simulink model "LKWDaempfungsModell"  (R2019b)
settings: Solver=VariableStepAuto  StartTime=0.0  StopTime=15  RelTol=1e-5
values from neighbouring files (symbols this model uses):
  F_FederRuhe = m_Frachtraum * g    (= 22563)    [modelParameter.m]
  g = 9.81    [modelParameter.m]
  K_Feder = 98.1 *1000    (= 98100)    [modelParameter.m]
  m_Frachtraum = 2300    [modelParameter.m]
  MaxActuatorForce = 100 *1000    (= 100000)    [modelParameter.m]
  muh_daempfer = 3000    [modelParameter.m]
libraries: simulink x1
settings Model: Creator=du-wa  LastModifiedBy=du-wa

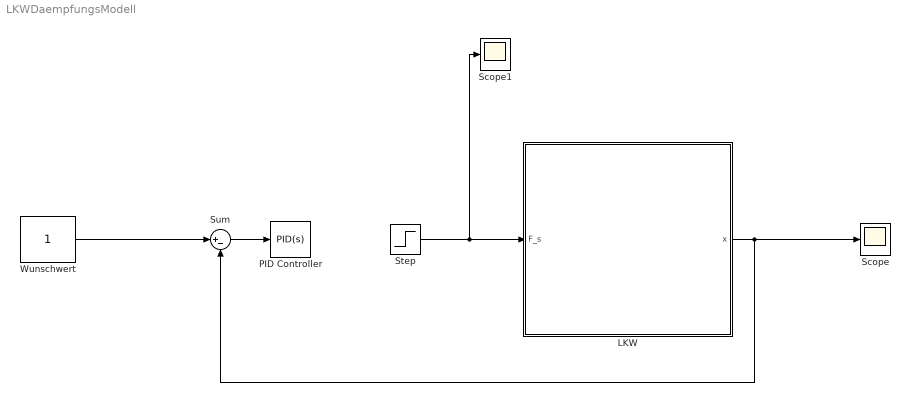
== system LKWDaempfungsModell ==
  "LKW " : Subsystem
  PID Controller : simulink/Continuous/PID Controller  Controller=PID  Form=Parallel  TimeDomain=Continuous-time  SampleTime=-1  IntegratorMethod=Forward Euler  FilterMethod=Forward Euler  ControllerParametersSource=internal  P=1000  I=1  D=0  UseFilter=on  N=100  TunerSelectOption=Transfer Function Based (PID Tuner App)  InitialConditionSource=internal  InitialConditionForIntegrator=0  InitialConditionForFilter=0  DifferentiatorICPrevScaledInput=0  ExternalReset=none  TrackingMode=off  Kt=1  LimitOutput=on  UpperSaturationLimit=MaxActuatorForce  LowerSaturationLimit=-MaxActuatorForce  LinearizeAsGain=on  AntiWindupMode=clamping  Kb=1  POutMin=[]  POutMax=[]  IOutMin=[]  IOutMax=[]  DOutMin=[]  DOutMax=[]  NOutMin=[]  NOutMax=[]  SumOutMin=[]  SumOutMax=[]  SaturationOutMin=[]  SaturationOutMax=[]  PParamMin=[]  PParamMax=[]  IParamMin=[]  IParamMax=[]  DParamMin=[]  DParamMax=[]  NParamMin=[]  NParamMax=[]  KbParamMin=[]  KbParamMax=[]  KtParamMin=[]  KtParamMax=[]  KbOutMin=[]  KbOutMax=[]  KtOutMin=[]  KtOutMax=[]  IntegratorOutMin=[]  IntegratorOutMax=[]  FilterOutMin=[]  FilterOutMax=[]  SumI1OutMin=[]  SumI1OutMax=[]  SumI2OutMin=[]  SumI2OutMax=[]  SumI3OutMin=[]  SumI3OutMax=[]  SumI4OutMin=[]  SumI4OutMax=[]  SumDOutMin=[]  SumDOutMax=[]  DifferentiatorOutMin=[]  DifferentiatorOutMax=[]  FilterDiffOutCoefMin=[]  FilterDiffOutCoefMax=[]  ReciprocalOutMin=[]  ReciprocalOutMax=[]  SumDenOutMin=[]  SumDenOutMax=[]  SumNumOutMin=[]  SumNumOutMax=[]  DivideOutMin=[]  DivideOutMax=[]  IntegratorContinuousStateAttributes=''  IntegratorStateMustResolveToSignalObject=off  IntegratorRTWStateStorageClass=Auto  FilterContinuousStateAttributes=''  FilterStateMustResolveToSignalObject=off  FilterRTWStateStorageClass=Auto  ParallelPVariant=InternalParameters  IdealPVariant=Disabled  IVariant=InternalParameters  DVariant=InternalParameters  IntegratorVariant=Continuous  SatVariant=Enabled  AWVariant=ContClampingParallel  PCopyVariant=Disabled  TRVariant=Disabled  FdbkBlocksVariant=Forward  IdealPFdbkVariant=Disabled  SatFdbkVariant=Disabled  DerivativeFilterVariant=ContFilter  NVariant=InternalParameters  NCopyVariant=Disabled  FilterICVariant=InternalICsFilter  IntegratorICVariant=InternalICs  ExternalResetVariant=Disabled  TRSumVariant=Passthrough  SumFdbkVariant=Disabled  SumVariant=Sum_PID
  Scope : Scope
  Scope1 : Scope
  Step : Step  After=1000  SampleTime=0
  Sum : Sum  Inputs=|+-
  Wunschwert : Constant
  wires:
  "LKW "/1(x) -> Scope/1, Sum/2
  Wunschwert/1 -> Sum/1
  Sum/1 -> PID Controller/1
  Step/1 -> Scope1/1, "LKW "/1(F_s)

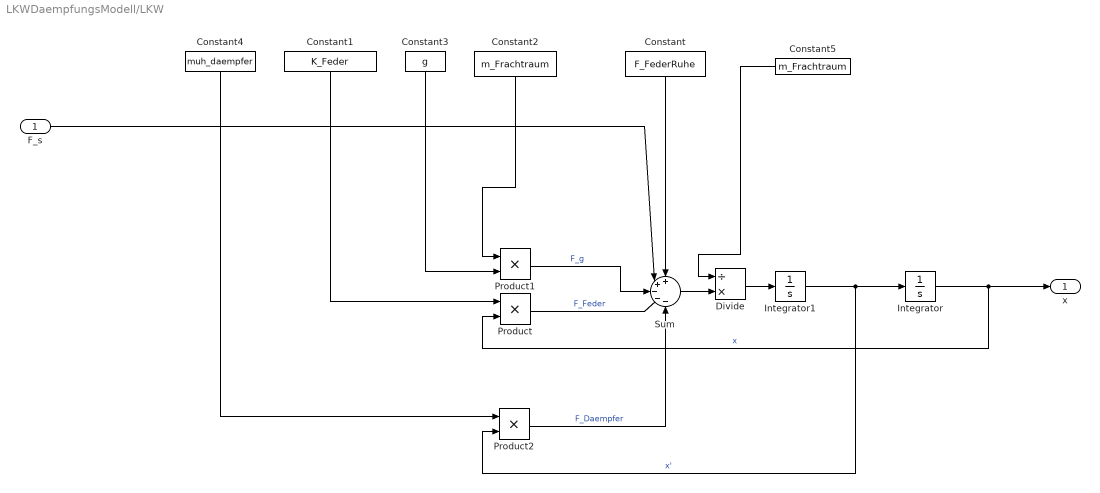
== system LKWDaempfungsModell/LKW  ==
  F_s : Inport
  Constant : Constant  Value=F_FederRuhe
  Constant1 : Constant  Value=K_Feder
  Constant2 : Constant  Value=m_Frachtraum
  Constant3 : Constant  Value=g
  Constant4 : Constant  Value=muh_daempfer
  Constant5 : Constant  Value=m_Frachtraum
  Divide : Product  Inputs=/*
  Integrator : Integrator
  Integrator1 : Integrator
  Product : Product
  Product1 : Product
  Product2 : Product
  Sum : Sum  Inputs=++---
  x : Outport
  wires:
  Constant1/1 -> Product/1
  Integrator1/1 -> Product2/2, Integrator/1  "x'"
  Constant4/1 -> Product2/1
  Constant/1 -> Sum/1
  Product1/1 -> Sum/3  "F_g"
  Constant2/1 -> Product1/1
  Integrator/1 -> x/1, Product/2  "x"
  Product2/1 -> Sum/5  "F_Daempfer"
  Product/1 -> Sum/4  "F_Feder"
  Constant3/1 -> Product1/2
  F_s/1 -> Sum/2
  Sum/1 -> Divide/2
  Constant5/1 -> Divide/1
  Divide/1 -> Integrator1/1
